simulink library "vehicle_dynamics_lib"  (R2022b)
settings: Solver=VariableStepAuto  StartTime=0.0  StopTime=10.0  RelTol=1e-3
libraries: $bdroot x1
settings Model: Creator=dr_pa  LastModifiedBy=LinF

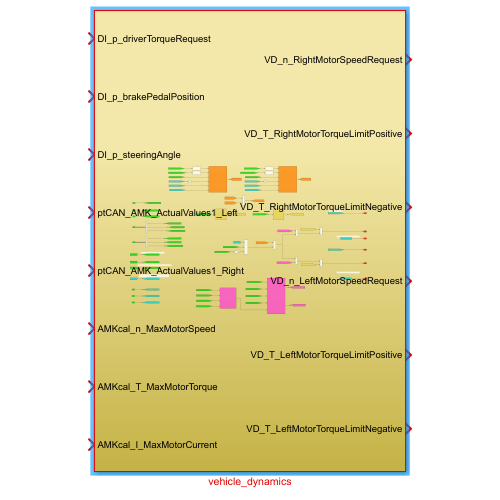
[thumbnail: Simulink's stored preview of the top-level diagram]
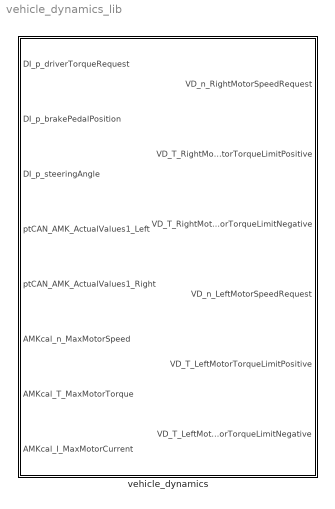
== system vehicle_dynamics_lib ==
  vehicle_dynamics : Subsystem

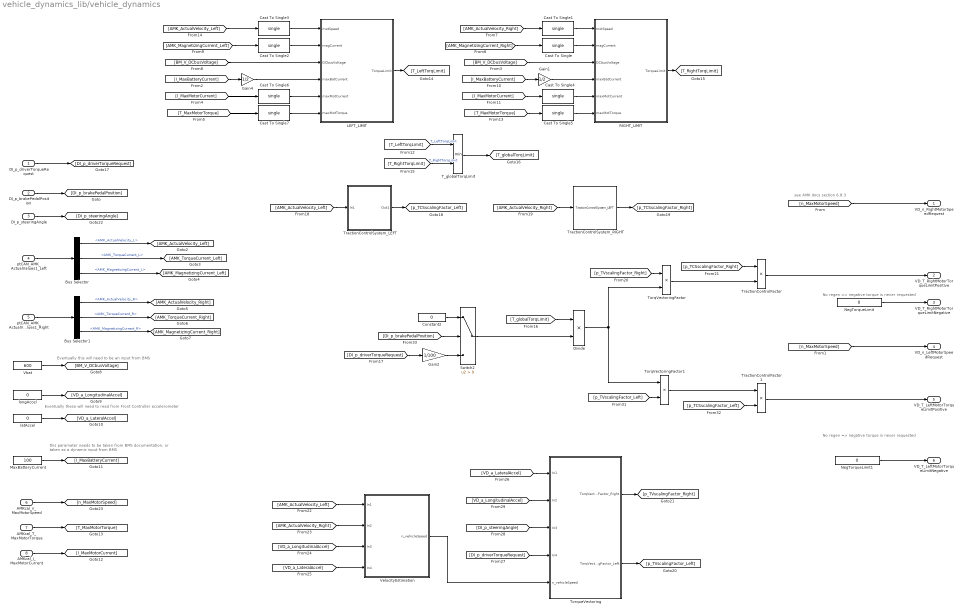
== system vehicle_dynamics_lib/vehicle_dynamics ==
  note: this parameter needs to be taken from BMS documentation, or
      | taken as a dynamic input from BMS
  note: Eventually this will need to be an input from BMS
  note: see AMK docs section 6.8.3
  note: No regen => negative torque is never requested
  note: No regen => negative torque is never requested
  note: Eventually these will need to read from Front Controller accelerometer
  DI_p_driverTorqueRequest : Inport
  DI_p_brakePedalPosition : Inport  Port=2
  DI_p_steeringAngle : Inport  Port=3
  ptCAN_AMK_ActualValues1_Left : Inport  Port=4
  ptCAN_AMK_ActualValues1_Right : Inport  Port=5
  AMKcal_n_MaxMotorSpeed : Inport  Port=6
  AMKcal_T_MaxMotorTorque : Inport  Port=7
  AMKcal_I_MaxMotorCurrent : Inport  Port=8
  Bus Selector : BusSelector  OutputSignals=AMK_ActualVelocity_L,AMK_TorqueCurrent_L,AMK_MagnetizingCurrent_L
  Bus Selector1 : BusSelector  OutputSignals=AMK_ActualVelocity_R,AMK_TorqueCurrent_R,AMK_MagnetizingCurrent_R
  Cast To Single{,1..7} (8 alike) : DataTypeConversion  OutDataTypeStr=single  SaturateOnIntegerOverflow=off  RndMeth=Floor
  Constant2 : Constant  Value=0  OutDataTypeStr=single
  Divide : Product  Inputs=**
  Gain1 : Gain  Gain=1/2
  Gain2 : Gain  Gain=1/100
  Gain4 : Gain  Gain=1/2
  LEFT_LIMIT : MATLAB Function  TreatAsAtomicUnit=on
  MaxBatteryCurrent : Constant  Value=100  OutDataTypeStr=single
  NegTorqueLimit : Constant  Value=0  OutDataTypeStr=single
  NegTorqueLimit1 : Constant  Value=0  OutDataTypeStr=single
  RIGHT_LIMIT : MATLAB Function  TreatAsAtomicUnit=on
  Switch2 : Switch  Criteria=u2 > Threshold  SaturateOnIntegerOverflow=off  InputSameDT=off
  T_globalTorqLimit : MinMax  Inputs=2
  TorqVectoringFactor : Product  Inputs=**
  TorqVectoringFactor1 : Product  Inputs=**
  TorqueVectoring : Subsystem
  TractionControlFactor : Product  Inputs=**
  TractionControlFactor1 : Product  Inputs=**
  TractionControlSystem_LEFT : Subsystem
  TractionControlSystem_RIGHT : $bdroot/vehicle_dynamics/TractionControlSystem_LEFT  SystemSampleTime=-1  VariantActivationTime=update diagram  Latency=0  AutoFrameSizeCalculation=off
  Vbat : Constant  Value=600  OutDataTypeStr=single
  VelocityEstimation : Subsystem
  latAccel : Constant  Value=0  OutDataTypeStr=single
  longAccel : Constant  Value=0  OutDataTypeStr=single
  VD_n_RightMotorSpeedRequest : Outport
  VD_T_RightMotorTorqueLimitPositive : Outport  Port=2
  VD_T_RightMotorTorqueLimitNegative : Outport  Port=3
  VD_n_LeftMotorSpeedRequest : Outport  Port=4
  VD_T_LeftMotorTorqueLimitPositive : Outport  Port=5
  VD_T_LeftMotorTorqueLimitNegative : Outport  Port=6
  wires:
  [n_MaxMotorSpeed] -> VD_n_RightMotorSpeedRequest/1
  NegTorqueLimit/1 -> VD_T_RightMotorTorqueLimitNegative/1
  [n_MaxMotorSpeed] -> VD_n_LeftMotorSpeedRequest/1
  NegTorqueLimit1/1 -> VD_T_LeftMotorTorqueLimitNegative/1
  ptCAN_AMK_ActualValues1_Right/1 -> Bus Selector1/1
  DI_p_steeringAngle/1 -> [DI_p_steeringAngle]
  DI_p_brakePedalPosition/1 -> [DI_p_brakePedalPosition]
  Bus Selector/1 -> [AMK_ActualVelocity_Left]  "<AMK_ActualVelocity_L>"
  Bus Selector/2 -> [AMK_TorqueCurrent_Left]  "<AMK_TorqueCurrent_L>"
  Vbat/1 -> [BM_V_DCbusVoltage]
  longAccel/1 -> [VD_a_LongitudinalAccel]
  latAccel/1 -> [VD_a_LateralAccel]
  [BM_V_DCbusVoltage] -> RIGHT_LIMIT/3(DCbusVoltage)
  [I_MaxBatteryCurrent] -> Gain1/1
  [I_MaxMotorCurrent] -> Cast To Single4/1
  MaxBatteryCurrent/1 -> [I_MaxBatteryCurrent]
  AMKcal_I_MaxMotorCurrent/1 -> [I_MaxMotorCurrent]
  Gain1/1 -> RIGHT_LIMIT/4(maxBatCurrent)
  AMKcal_T_MaxMotorTorque/1 -> [T_MaxMotorTorque]
  [T_MaxMotorTorque] -> Cast To Single5/1
  RIGHT_LIMIT/1(TorqueLimit) -> [T_RightTorqLimit]
  [T_LeftTorqLimit] -> T_globalTorqLimit/1  "T_LeftTorqLimit"
  [T_RightTorqLimit] -> T_globalTorqLimit/2  "T_RightTorqLimit"
  T_globalTorqLimit/1 -> [T_globalTorqLimit]
  DI_p_driverTorqueRequest/1 -> [DI_p_driverTorqueRequest]
  [DI_p_driverTorqueRequest] -> Gain2/1
  [AMK_ActualVelocity_Left] -> TractionControlSystem_LEFT/1(In1)
  [AMK_ActualVelocity_Right] -> TractionControlSystem_RIGHT/1
  TractionControlSystem_LEFT/1(Out1) -> [p_TCSscalingFactor_Left]
  TractionControlSystem_RIGHT/1 -> [p_TCSscalingFactor_Right]
  [p_TCSscalingFactor_Right] -> TractionControlFactor/1
  TorqVectoringFactor/1 -> TractionControlFactor/2
  Divide/1 -> TorqVectoringFactor/2, TorqVectoringFactor1/1
  TorqueVectoring/2(TorqVectoringFactor_Left) -> [p_TVscalingFactor_Left]
  TorqueVectoring/1(TorqVectoringFactor_Right) -> [p_TVscalingFactor_Right]
  [p_TVscalingFactor_Right] -> TorqVectoringFactor/1
  [AMK_ActualVelocity_Left] -> VelocityEstimation/1(In1)
  [AMK_ActualVelocity_Right] -> VelocityEstimation/2(In2)
  [VD_a_LongitudinalAccel] -> VelocityEstimation/3(In3)
  [VD_a_LateralAccel] -> VelocityEstimation/4(In4)
  [VD_a_LateralAccel] -> TorqueVectoring/1(In1)
  [VD_a_LongitudinalAccel] -> TorqueVectoring/2(In2)
  [DI_p_steeringAngle] -> TorqueVectoring/3(In3)
  [DI_p_driverTorqueRequest] -> TorqueVectoring/4(In4)
  VelocityEstimation/1(n_vehicleSpeed) -> TorqueVectoring/5(n_vehicleSpeed)
  Bus Selector/3 -> [AMK_MagnetizingCurrent_Left]  "<AMK_MagnetizingCurrent_L>"
  Bus Selector1/2 -> [AMK_TorqueCurrent_Right]  "<AMK_TorqueCurrent_R>"
  Bus Selector1/3 -> [AMK_MagnetizingCurrent_Right]  "<AMK_MagnetizingCurrent_R>"
  TractionControlFactor/1 -> VD_T_RightMotorTorqueLimitPositive/1
  LEFT_LIMIT/1(TorqueLimit) -> [T_LeftTorqLimit]
  Bus Selector1/1 -> [AMK_ActualVelocity_Right]  "<AMK_ActualVelocity_R>"
  Gain2/1 -> Switch2/3
  ptCAN_AMK_ActualValues1_Left/1 -> Bus Selector/1
  [T_MaxMotorTorque] -> Cast To Single7/1
  [I_MaxMotorCurrent] -> Cast To Single6/1
  [I_MaxBatteryCurrent] -> Gain4/1
  Gain4/1 -> LEFT_LIMIT/4(maxBatCurrent)
  [BM_V_DCbusVoltage] -> LEFT_LIMIT/3(DCbusVoltage)
  AMKcal_n_MaxMotorSpeed/1 -> [n_MaxMotorSpeed]
  [DI_p_brakePedalPosition] -> Switch2/2
  Constant2/1 -> Switch2/1
  Switch2/1 -> Divide/2
  [T_globalTorqLimit] -> Divide/1
  TractionControlFactor1/1 -> VD_T_LeftMotorTorqueLimitPositive/1
  [p_TCSscalingFactor_Left] -> TractionControlFactor1/2
  TorqVectoringFactor1/1 -> TractionControlFactor1/1
  [p_TVscalingFactor_Left] -> TorqVectoringFactor1/2
  [AMK_MagnetizingCurrent_Right] -> Cast To Single/1
  Cast To Single/1 -> RIGHT_LIMIT/2(magCurrent)
  [AMK_ActualVelocity_Right] -> Cast To Single1/1
  Cast To Single1/1 -> RIGHT_LIMIT/1(motSpeed)
  [AMK_ActualVelocity_Left] -> Cast To Single3/1
  Cast To Single3/1 -> LEFT_LIMIT/1(motSpeed)
  [AMK_MagnetizingCurrent_Left] -> Cast To Single2/1
  Cast To Single2/1 -> LEFT_LIMIT/2(magCurrent)
  Cast To Single4/1 -> RIGHT_LIMIT/5(maxMotCurrent)
  Cast To Single5/1 -> RIGHT_LIMIT/6(maxMotTorque)
  Cast To Single6/1 -> LEFT_LIMIT/5(maxMotCurrent)
  Cast To Single7/1 -> LEFT_LIMIT/6(maxMotTorque)

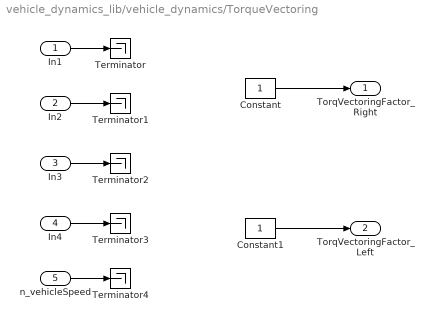
== system vehicle_dynamics_lib/vehicle_dynamics/TorqueVectoring ==
  In1 : Inport
  In2 : Inport  Port=2
  In3 : Inport  Port=3
  In4 : Inport  Port=4
  n_vehicleSpeed : Inport  Port=5
  Constant : Constant  OutDataTypeStr=single
  Constant1 : Constant  OutDataTypeStr=single
  Terminator{,1..4} (5 alike) : Terminator
  TorqVectoringFactor_Right : Outport
  TorqVectoringFactor_Left : Outport  Port=2
  wires:
  Constant1/1 -> TorqVectoringFactor_Left/1
  Constant/1 -> TorqVectoringFactor_Right/1
  In1/1 -> Terminator/1
  In2/1 -> Terminator1/1
  In3/1 -> Terminator2/1
  In4/1 -> Terminator3/1
  n_vehicleSpeed/1 -> Terminator4/1

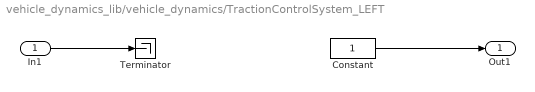
== system vehicle_dynamics_lib/vehicle_dynamics/TractionControlSystem_LEFT ==
  In1 : Inport
  Constant : Constant  OutDataTypeStr=single
  Terminator : Terminator
  Out1 : Outport
  wires:
  In1/1 -> Terminator/1
  Constant/1 -> Out1/1

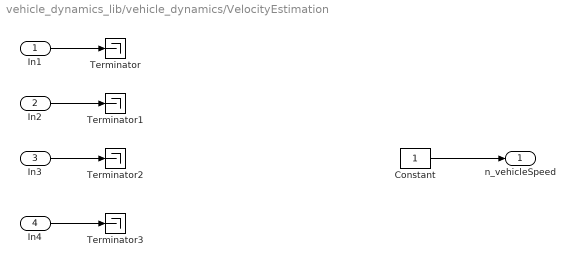
== system vehicle_dynamics_lib/vehicle_dynamics/VelocityEstimation ==
  In1 : Inport
  In2 : Inport  Port=2
  In3 : Inport  Port=3
  In4 : Inport  Port=4
  Constant : Constant  OutDataTypeStr=single
  Terminator{,1..3} (4 alike) : Terminator
  n_vehicleSpeed : Outport
  wires:
  Constant/1 -> n_vehicleSpeed/1
  In1/1 -> Terminator/1
  In2/1 -> Terminator1/1
  In3/1 -> Terminator2/1
  In4/1 -> Terminator3/1

== matlab function vehicle_dynamics_lib/vehicle_dynamics/RIGHT_LIMIT ==
  data: motSpeed input single; TorqueLimit output single; magCurrent input single; DCbusVoltage input single; maxBatCurrent input single; maxMotCurrent input single; maxMotTorque input
function TorqueLimit = MaxAvailableTorque(motSpeed, magCurrent, DCbusVoltage ,maxBatCurrent, maxMotCurrent, maxMotTorque)

% this function computes the motor's available torque based solely on it's 
% available power (limited by max current and DC voltage). It does not account for
% over-temperature torque limitation

magCurrent = max(magCurrent,0); % saturate below 0
globalCurrentLimit = min(maxBatCurrent,maxMotCurrent);
motSpeed = max(motSpeed,1); % saturate below 1rpm (avoid divide-by-0)

% rearranged from I_total = I_torq^2 + I_mag^2 < I_limit^2
% see AMK docs pg 36
availableTorqCurrent = max(sqrt(globalCurrentLimit^2 - magCurrent^2), 0); % saturate below 0

% solve for Torq in Torq*speed = Volts*Amps
TorqueLimit = availableTorqCurrent * DCbusVoltage / (motSpeed * pi/30); % convert motSpeed from rpm to rad/s

% saturate above by rated peak torque, below by 0
TorqueLimit = min(max(TorqueLimit,0),maxMotTorque);

== matlab function vehicle_dynamics_lib/vehicle_dynamics/LEFT_LIMIT ==
  data: motSpeed input single; TorqueLimit output single; magCurrent input single; DCbusVoltage input single; maxBatCurrent input single; maxMotCurrent input single; maxMotTorque input
function TorqueLimit = MaxAvailableTorque(motSpeed, magCurrent, DCbusVoltage ,maxBatCurrent, maxMotCurrent, maxMotTorque)

% this function computes the motor's available torque based solely on it's 
% available power (limited by max current and DC voltage). It does not account for
% over-temperature torque limitation

magCurrent = max(magCurrent,0); % saturate below 0
globalCurrentLimit = min(maxBatCurrent,maxMotCurrent);
motSpeed = max(motSpeed,1); % saturate below 1rpm (avoid divide-by-0)

% rearranged from I_total = I_torq^2 + I_mag^2 < I_limit^2
% see AMK docs pg 36
availableTorqCurrent = max(sqrt(globalCurrentLimit^2 - magCurrent^2), 0); % saturate below 0

% solve for Torq in Torq*speed = Volts*Amps
TorqueLimit = availableTorqCurrent * DCbusVoltage / (motSpeed * pi/30); % convert motSpeed from rpm to rad/s

% saturate above by rated peak torque, below by 0
TorqueLimit = min(max(TorqueLimit,0),maxMotTorque);
